simulink model "model"  (R2015a)
settings: Solver=ode45  StartTime=0.0  StopTime=50  RelTol=1e-3
values from neighbouring files (symbols this model uses):
  den = G.den{1,1}    [main.m]
  K = 0.95/a    [aproksymacja.m]    (also in main.m = 0.6/a)
  num = G.num{1,1}    [main.m]
  Td = 0.42*L    [aproksymacja.m]    (also in main.m = 0.5*L)
  Ti = 2.4*L    [aproksymacja.m]    (also in main.m = 1.0*T_p)
libraries: simulink x1
settings Model: Creator=Warzyn  LastModifiedBy=Warzyn

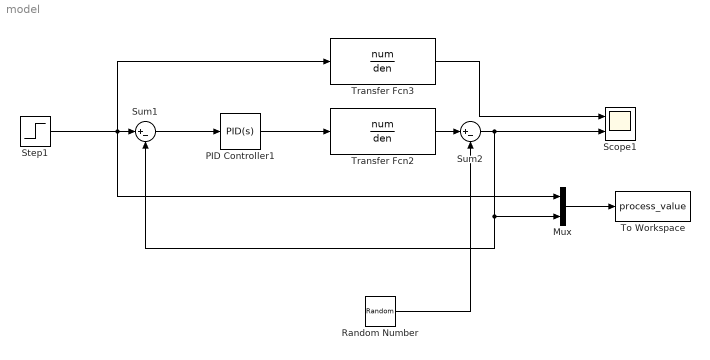
== system model ==
  Mux : Mux  Inputs=2
  PID Controller1 : simulink/Continuous/PID Controller  Controller=PID  TimeDomain=Continuous-time  SampleTime=-1  IntegratorMethod=Forward Euler  FilterMethod=Forward Euler  Form=Ideal  UseFilter=on  ControllerParametersSource=internal  P=K  I=Ti  D=Td  N=1  InitialConditionSource=internal  InitialConditionForIntegrator=0  InitialConditionForFilter=0  ExternalReset=none  LimitOutput=off  UpperSaturationLimit=inf  LowerSaturationLimit=-inf  LinearizeAsGain=on  AntiWindupMode=none  Kb=1  TrackingMode=off  Kt=1  PParamMin=[]  PParamMax=[]  IParamMin=[]  IParamMax=[]  DParamMin=[]  DParamMax=[]  NParamMin=[]  NParamMax=[]  KbParamMin=[]  KbParamMax=[]  KtParamMin=[]  KtParamMax=[]  POutMin=[]  POutMax=[]  IOutMin=[]  IOutMax=[]  DOutMin=[]  DOutMax=[]  NOutMin=[]  NOutMax=[]  KbOutMin=[]  KbOutMax=[]  KtOutMin=[]  KtOutMax=[]  IntegratorOutMin=[]  IntegratorOutMax=[]  FilterOutMin=[]  FilterOutMax=[]  SumOutMin=[]  SumOutMax=[]  SumI1OutMin=[]  SumI1OutMax=[]  SumI2OutMin=[]  SumI2OutMax=[]  SumI3OutMin=[]  SumI3OutMax=[]  SumDOutMin=[]  SumDOutMax=[]  SaturationOutMin=[]  SaturationOutMax=[]  IntegratorContinuousStateAttributes=''  IntegratorStateMustResolveToSignalObject=off  IntegratorRTWStateStorageClass=Auto  FilterContinuousStateAttributes=''  FilterStateMustResolveToSignalObject=off  FilterRTWStateStorageClass=Auto  DifferentiatorICPrevScaledInput=0  DifferentiatorOutMin=[]  DifferentiatorOutMax=[]
  Random Number : RandomNumber  Variance=0  SampleTime=0.1
  Scope1 : Scope  NumInputPorts=2
      settings: YMin=-2.0881e-53~-5  YMax=1e-36~5
  Step1 : Step  After=2  SampleTime=0
  Sum1 : Sum  Inputs=|+-
  Sum2 : Sum  Inputs=|+-
  To Workspace : ToWorkspace  VariableName=process_value  SaveFormat=Structure With Time  SampleTime=-1
  Transfer Fcn2 : TransferFcn  Numerator=num  Denominator=den
  Transfer Fcn3 : TransferFcn  Numerator=num  Denominator=den
  wires:
  Sum1/1 -> PID Controller1/1
  PID Controller1/1 -> Transfer Fcn2/1
  Transfer Fcn3/1 -> Scope1/1
  Step1/1 -> Mux/1, Transfer Fcn3/1, Sum1/1
  Mux/1 -> To Workspace/1
  Transfer Fcn2/1 -> Sum2/1
  Random Number/1 -> Sum2/2
  Sum2/1 -> Mux/2, Sum1/2, Scope1/2
